simulink model "fw_mixer_output"  (R2024b)
settings: Solver=FixedStepAuto  StartTime=0.0  StopTime=10.0  FixedStep=0.005  RelTol=1e-3
settings Model: DataDictionary=nextpilot_datadict.sldd  Creator=CETCA  LastModifiedBy=CETCA

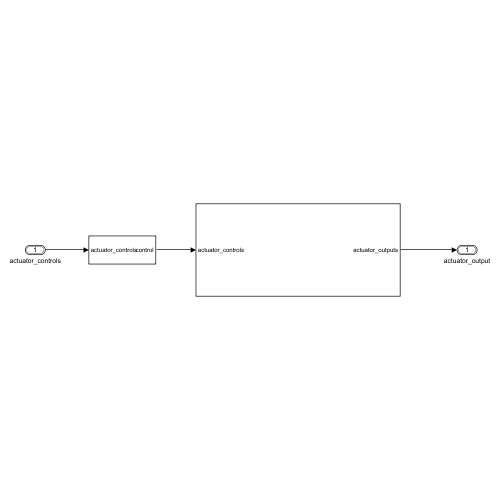
[thumbnail: Simulink's stored preview of the top-level diagram]
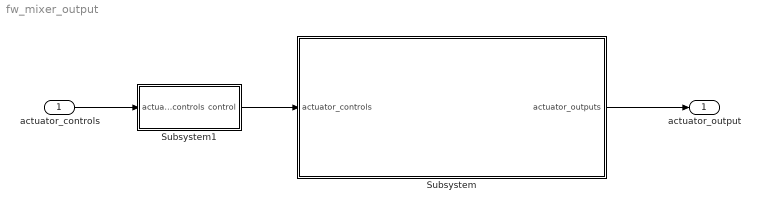
== system fw_mixer_output ==
  actuator_controls : Inport  OutDataTypeStr=Bus: actuator_controls_s
  Subsystem : Subsystem
  Subsystem1 : Subsystem
  actuator_output : Outport  OutDataTypeStr=Bus: actuator_outputs_s
  wires:
  actuator_controls/1 -> Subsystem1/1(actuator_controls)
  Subsystem/1(actuator_outputs) -> actuator_output/1
  Subsystem1/1(control) -> Subsystem/1(actuator_controls)

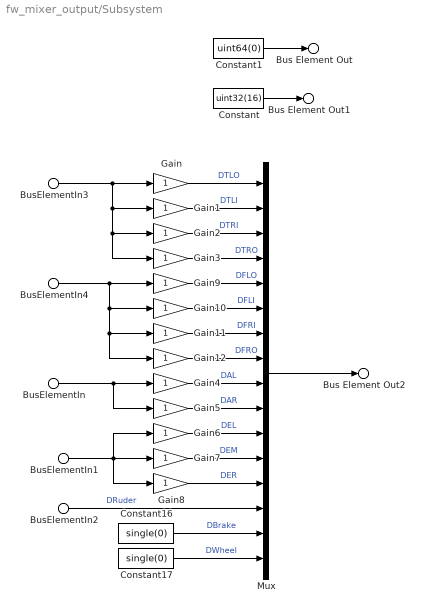
== system fw_mixer_output/Subsystem ==
  BusElementIn : Inport  PortName=actuator_controls  Element=roll
  BusElementIn1 : Inport  PortName=actuator_controls  Element=pitch
  BusElementIn2 : Inport  PortName=actuator_controls  Element=yaw
  BusElementIn3 : Inport  PortName=actuator_controls  Element=throttle
  BusElementIn4 : Inport  PortName=actuator_controls  Element=flaps
  Constant : Constant  Value=uint32(16)
  Constant1 : Constant  Value=uint64(0)
  Constant16 : Constant  Value=single(0)
  Constant17 : Constant  Value=single(0)
  Gain{,1..12} (13 alike) : Gain
  Mux : Mux  Inputs=16
  Bus Element Out : Outport  PortName=actuator_outputs  Element=timestamp
  Bus Element Out1 : Outport  PortName=actuator_outputs  Element=noutputs
  Bus Element Out2 : Outport  PortName=actuator_outputs  Element=output
  wires:
  Constant/1 -> Bus Element Out1/1
  Constant1/1 -> Bus Element Out/1
  Mux/1 -> Bus Element Out2/1
  BusElementIn3/1 -> Gain1/1, Gain2/1, Gain3/1, Gain/1
  Gain1/1 -> Mux/2  "DTLI"
  Gain2/1 -> Mux/3  "DTRI"
  Gain3/1 -> Mux/4  "DTRO"
  BusElementIn4/1 -> Gain9/1, Gain10/1, Gain11/1, Gain12/1
  BusElementIn/1 -> Gain4/1, Gain5/1
  BusElementIn1/1 -> Gain7/1, Gain8/1, Gain6/1
  BusElementIn2/1 -> Mux/14  "DRuder"
  Constant16/1 -> Mux/15  "DBrake"
  Constant17/1 -> Mux/16  "DWheel"
  Gain/1 -> Mux/1  "DTLO"
  Gain4/1 -> Mux/9  "DAL"
  Gain5/1 -> Mux/10  "DAR"
  Gain6/1 -> Mux/11  "DEL"
  Gain7/1 -> Mux/12  "DEM"
  Gain8/1 -> Mux/13  "DER"
  Gain9/1 -> Mux/5  "DFLO"
  Gain10/1 -> Mux/6  "DFLI"
  Gain11/1 -> Mux/7  "DFRI"
  Gain12/1 -> Mux/8  "DFRO"

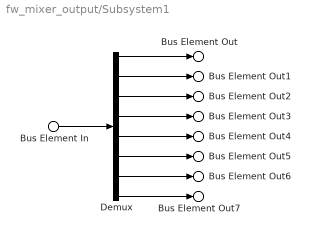
== system fw_mixer_output/Subsystem1 ==
  Bus Element In : Inport  PortName=actuator_controls  Element=control
  Demux : Demux  Outputs=8
  Bus Element Out : Outport  PortName=control  Element=roll
  Bus Element Out1 : Outport  PortName=control  Element=pitch
  Bus Element Out2 : Outport  PortName=control  Element=yaw
  Bus Element Out3 : Outport  PortName=control  Element=throttle
  Bus Element Out4 : Outport  PortName=control  Element=flaps
  Bus Element Out5 : Outport  PortName=control  Element=spoilers
  Bus Element Out6 : Outport  PortName=control  Element=airbrakes
  Bus Element Out7 : Outport  PortName=control  Element=landgear
  wires:
  Bus Element In/1 -> Demux/1
  Demux/1 -> Bus Element Out/1
  Demux/2 -> Bus Element Out1/1
  Demux/3 -> Bus Element Out2/1
  Demux/4 -> Bus Element Out3/1
  Demux/5 -> Bus Element Out4/1
  Demux/6 -> Bus Element Out5/1
  Demux/7 -> Bus Element Out6/1
  Demux/8 -> Bus Element Out7/1
